simulink model "Phasor"  (Simulink 7.9)
settings: Solver=FixedStepDiscrete  StartTime=0.0  StopTime=Inf  FixedStep=0.0001  RelTol=1e-3
libraries: simulink x3
settings Model: Creator=DBR  LastModifiedBy=DBR

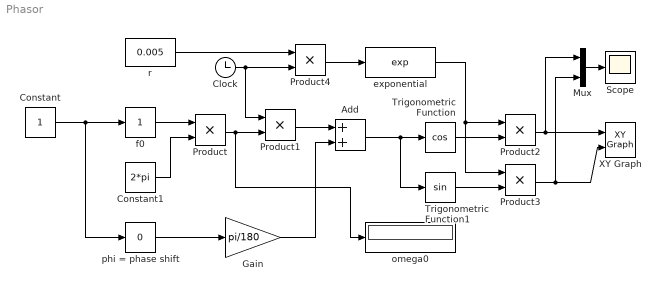
== system Phasor ==
  Add : Sum
  Clock : Clock
  Constant : Constant
  Constant1 : Constant  Value=2*pi
  Gain : Gain  Gain=pi/180
  Mux : Mux  Inputs=2
  Product{,1..4} (5 alike) : Product  RndMeth=Zero
  Scope : Scope
      settings: TimeRange=5  YMin=-1.5  YMax=1.5
  Trigonometric Function : Trigonometry  Operator=cos
  Trigonometric Function1 : Trigonometry
  XY Graph : simulink/Sinks/XY Graph  xmin=-1.1  xmax=1.1  ymin=-1.1  ymax=1.1  st=-1
  exponential : MATLABFcn  MATLABFcn=exp
  f0 : simulink/Math Operations/Slider Gain  low=1  gain=1  high=10
  omega0 : Display
  phi = phase shift : simulink/Math Operations/Slider Gain  low=-180  gain=0  high=180
  r : Constant  Value=0.005
  wires:
  Constant/1 -> f0/1, phi = phase shift/1
  f0/1 -> Product/1
  Constant1/1 -> Product/2
  Add/1 -> Trigonometric Function/1, Trigonometric Function1/1
  Product/1 -> Product1/2, omega0/1
  Clock/1 -> Product4/2, Product1/1
  Product1/1 -> Add/1
  Trigonometric Function/1 -> Product2/2
  Trigonometric Function1/1 -> Product3/2
  Product2/1 -> XY Graph/1, Mux/1
  r/1 -> Product4/1
  exponential/1 -> Product2/1, Product3/1
  Product3/1 -> XY Graph/2, Mux/2
  phi = phase shift/1 -> Gain/1
  Gain/1 -> Add/2
  Product4/1 -> exponential/1
  Mux/1 -> Scope/1
